simulink model "mod"  (R2019a)
settings: Solver=VariableStepAuto  StartTime=0  StopTime=1369  RelTol=1e-3
undefined symbols (not defined in the file): Ion, Lithium
libraries: nesl_utility x7, fl_lib x6, sdl_lib x5, autolibshared x4, ee_lib x3, powerlib x2, electricdrivelib x1
settings Model: SnapshotBufferSize=50  Creator=rachad  LastModifiedBy=rachad
settings GRTTargetCC: ExtMode=on

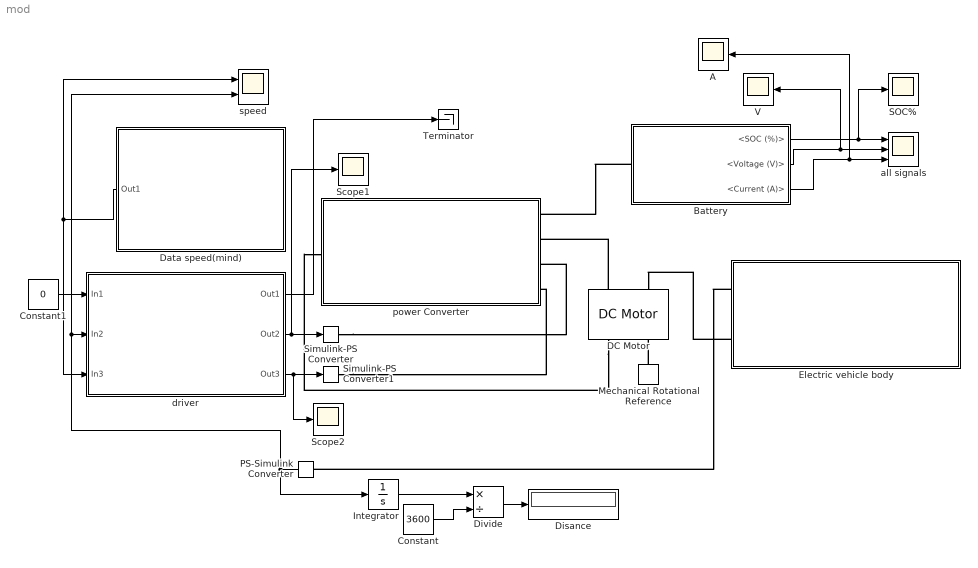
== system mod ==
  A : Scope
  Battery : Subsystem
  Constant : Constant  Value=3600
  Constant1 : Constant  Value=0
  DC Motor : ee_lib/Electromechanical/Brushed Motors/DC Motor  parameterization=3  Ra=3.9 Ohm  La=12e-6 H  emf_or_torque=1  Kv=0.072e-3 V/rpm  Ki=6.876e-4 N*m/A  T_stall=0.24e-3 N*m  w_max=15000 rpm  w_rated=12000 rpm  P_rated=150 kW  V_rated=300 V  J=0.01 g*cm^2  lam_param=1  lam=0 N*m/(rad/s)  i_noload=0 A  V_i_noload=1.5 V  speed0=0 rpm  alpha=3.93e-3 1/K  Tmeas=25 degC  thermal_mass=100 J/K  initial_temperature=25 degC
      settings: SourceProductName=Simscape Electrical
  Data speed(mind) : Subsystem
  Disance : Display
  Divide : Product  Inputs=*/
  Electric vehicle body : Subsystem
  Integrator : Integrator
  Mechanical Rotational Reference : fl_lib/Mechanical/Rotational Elements/Mechanical Rotational Reference
  PS-Simulink Converter : nesl_utility/PS-Simulink Converter  PhysicalDomain=network_engine_domain  SubClassName=ps_output  LeftPortType=input  RightPortType=output  PseudoPeriodic=off  Frequencies=[]  Unit=m/s  AffineConversion=off
  SOC% : Scope
  Scope1 : Scope
  Scope2 : Scope
  Simulink-PS Converter : nesl_utility/Simulink-PS Converter  PhysicalDomain=network_engine_domain  SubClassName=ps_input  LeftPortType=input  RightPortType=output  PseudoPeriodic=off  Frequencies=[]  NoiseDistribution=none  NoiseParameters=[]  Unit=1  AffineConversion=off  FilteringAndDerivatives=provide  SimscapeFilterOrder=1  InputFilterTimeConstant=0.001  UdotUserProvided=0
  Simulink-PS Converter1 : nesl_utility/Simulink-PS Converter  PhysicalDomain=network_engine_domain  SubClassName=ps_input  LeftPortType=input  RightPortType=output  PseudoPeriodic=off  Frequencies=[]  NoiseDistribution=none  NoiseParameters=[]  Unit=1  AffineConversion=off  FilteringAndDerivatives=provide  SimscapeFilterOrder=1  InputFilterTimeConstant=0.001  UdotUserProvided=0
  Terminator : Terminator
  V : Scope
  all signals : Scope  NumInputPorts=3
  driver : Subsystem
  power Converter : Subsystem
  speed : Scope  NumInputPorts=2
  wires:
  Divide/1 -> Disance/1
  Constant/1 -> Divide/2
  Integrator/1 -> Divide/1
  driver/2(Out2) -> Simulink-PS Converter/1, Scope1/1
  Constant1/1 -> driver/1(In1)
  driver/3(Out3) -> Simulink-PS Converter1/1, Scope2/1
  Data speed(mind)/1(Out1) -> speed/1, driver/3(In3)
  Battery/1(<SOC (%)>) -> SOC%/1, all signals/1
  Battery/2(<Voltage (V)>) -> V/1, all signals/2
  Battery/3(<Current (A)>) -> A/1, all signals/3
  PS-Simulink Converter/1 -> speed/2, driver/2(In2), Integrator/1
  driver/1(Out1) -> Terminator/1
  connections:
  Electric vehicle body/LConn2 -- DC Motor/LConn2
  Mechanical Rotational Reference/LConn1 -- DC Motor/RConn2
  Electric vehicle body/LConn1 -- PS-Simulink Converter/LConn1
  DC Motor/LConn1 -- power Converter/RConn2
  DC Motor/RConn1 -- power Converter/LConn1
  Simulink-PS Converter/RConn1 -- power Converter/RConn3
  Simulink-PS Converter1/RConn1 -- power Converter/RConn4
  Battery/LConn1 -- power Converter/RConn1

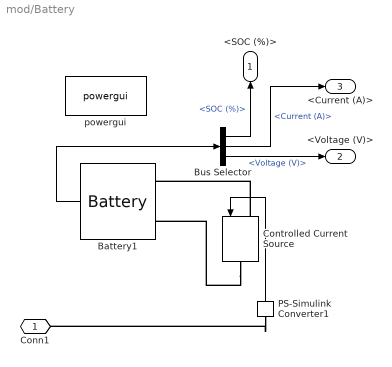
== system mod/Battery ==
  Battery1 : electricdrivelib/Extra Sources/Battery  BatType=Lithium-Ion  ShowTempParam=off  ThermalPreset=no  ShowAgeParam=off  NomV=300  NomQ=50  SOC=100  Batt_Tr=1  PresetModel=on  MaxQ=50  MinV=225  FullV=349.1961  Dis_rate=21.7391  R=0.06  Normal_OP=45.2174  expZone="[324.1158      2.456522]"  current=[6.5 13 32.5]  Units=Time  Tci=20  NomT=20  T2=-30  MaxQ2=4.8  FullV2=7.1  Normal_OP2=5.655  expZone2="[6.58           1]"  Rca=0.6  ti=2000  Dp=0  Neq0=0  Tsim=1e6  Ta1=25  Qeol=5.4*0.9  Reol=0.013333*1.2  Char_age=[2.3478, 3]  Dis_age=[2.3478, 10]  N1=1500  N2=10500  N3=1000  N4=1400  Ta2=45  N5=950
      settings: SourceProductName=Simscape Electrical
  Bus Selector : BusSelector  OutputSignals=SOC (%),Current (A),Voltage (V)
  Controlled Current Source : powerlib/Electrical Sources/Controlled Current Source  Initialize=off  Source_Type=DC  Amplitude=0  Phase=0  Frequency=0  Measurements=None
      settings: SourceProductName=Simscape Electrical
  PS-Simulink Converter1 : nesl_utility/PS-Simulink Converter  PhysicalDomain=network_engine_domain  SubClassName=ps_output  LeftPortType=input  RightPortType=output  PseudoPeriodic=off  Frequencies=[]  Unit=1  AffineConversion=off
  powergui : powerlib/powergui  Priority=1  SimulationMode=Continuous  SampleTime=50e-6  frequency=60  Iterations=50  frequencyindice=0  Pbase=100e6  ErrMax=1e-4  UnitsV=kV  UnitsW=MW  buscounter=0  FunctionMessages=off  echomessages=off  EnableUseOfTLC=off  CurrentSourceSwitches=off  DisableSnubberDevices=off  DisableRonSwitches=off  DisableVfSwitches=off  DisplayEquations=off  AutomaticDiscreteSolvers=off  SolverType=Tustin/Backward Euler (TBE)  Interpol=off  ExternalGateDelay=off  methode=off  Ts=100  x0status=blocks  SPID=on  SwTol=0  HookPort=off  NonlinearTolerance=0  nMaxIteration=15  ContinueOnMaxIteration=off  RestoreLinks=warning  ResistiveCurrentMeasurement=off  Frange=[0:2:500]  Ylog=off  Xlog=on  ShowGrid=off  save=off  variable=ZData  structure=0  ZoomFFT=off  StartTime=0.0  cycles=1  DisplayStyle=1  fundamental=60  FreqAxis=off  MaxFrequency=1000  frequencyindicesteady=1  RmsSteady=1  display=off
      settings: SourceProductName=Simscape Electrical
  Conn1 : PMIOPort  Side=Left
  <SOC (%)> : Outport
  <Voltage (V)> : Outport  Port=2
  <Current (A)> : Outport  Port=3
  wires:
  Bus Selector/2 -> <Current (A)>/1  "<Current (A)>"
  Bus Selector/3 -> <Voltage (V)>/1  "<Voltage (V)>"
  PS-Simulink Converter1/1 -> Controlled Current Source/1
  Battery1/1 -> Bus Selector/1
  Bus Selector/1 -> <SOC (%)>/1  "<SOC (%)>"
  connections:
  Controlled Current Source/LConn1 -- Battery1/LConn1
  Controlled Current Source/RConn1 -- Battery1/LConn2
  PS-Simulink Converter1/LConn1 -- Conn1/RConn1

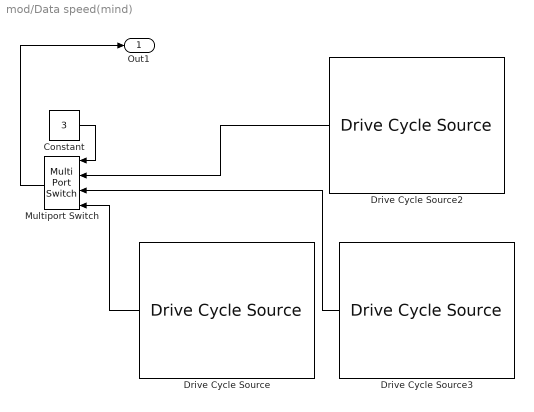
== system mod/Data speed(mind) ==
  Constant : Constant  Value=3
  Drive Cycle Source : autolibshared/Drive Cycle Source  cycleVar=.mat, .xls, .xlsx or .txt file  fileVar=C:\Users\rachad\Desktop\udds.txt  tfinal="1369  seconds"  cycleRepeat=off  outAccPort=off  outGearPort=off  gearList=No gear data  t_wot1=5  xdot_woto=0  xdot_wot1=30  t_wot2=20  xdot_wot2=0  t_wotend=30  srcUnit=m/s  outUnit=m/s  srcAccUnit=m/s/s  outAccUnit=m/s^2  dt=0  aMode=1
      settings: SourceProductName=Powertrain Blockset  SourceProductBaseCode=PW
  Drive Cycle Source2 : autolibshared/Drive Cycle Source  cycleVar=FTP75  fileVar=cycleFTP75.mat  tfinal="2474  seconds"  cycleRepeat=off  outAccPort=off  outGearPort=off  gearList=No gear data  t_wot1=5  xdot_woto=0  xdot_wot1=30  t_wot2=20  xdot_wot2=0  t_wotend=30  srcUnit=m/s  outUnit=m/s  srcAccUnit=m/s/s  outAccUnit=m/s^2  dt=0  aMode=1
      settings: SourceProductName=Powertrain Blockset  SourceProductBaseCode=PW
  Drive Cycle Source3 : autolibshared/Drive Cycle Source  cycleVar=.mat, .xls, .xlsx or .txt file  fileVar=C:\Users\rachad\Desktop\IM240.txt  tfinal="240  seconds"  cycleRepeat=off  outAccPort=off  outGearPort=off  gearList=No gear data  t_wot1=5  xdot_woto=0  xdot_wot1=30  t_wot2=20  xdot_wot2=0  t_wotend=30  srcUnit=m/s  outUnit=m/s  srcAccUnit=m/s/s  outAccUnit=m/s^2  dt=0  aMode=1
      settings: SourceProductName=Powertrain Blockset  SourceProductBaseCode=PW
  Multiport Switch : MultiPortSwitch
  Out1 : Outport
  wires:
  Multiport Switch/1 -> Out1/1
  Drive Cycle Source/1 -> Multiport Switch/4
  Constant/1 -> Multiport Switch/1
  Drive Cycle Source2/1 -> Multiport Switch/2
  Drive Cycle Source3/1 -> Multiport Switch/3

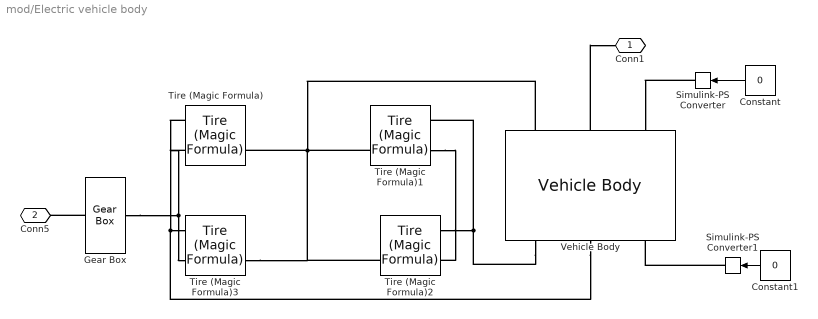
== system mod/Electric vehicle body ==
  Constant : Constant  Value=0
  Constant1 : Constant  Value=0
  Gear Box : fl_lib/Mechanical/Mechanisms/Gear Box  ratio=7  t_in_specify=off  t_in_priority=None  t_in=0 N*m  t_in_nominal_specify=off  t_in_nominal_unit=N*m  t_in_nominal_value=1  t_out_specify=off  t_out_priority=None  t_out=0 N*m  t_out_nominal_specify=off  t_out_nominal_unit=N*m  t_out_nominal_value=1
  Simulink-PS Converter : nesl_utility/Simulink-PS Converter  PhysicalDomain=network_engine_domain  SubClassName=ps_input  LeftPortType=input  RightPortType=output  PseudoPeriodic=off  Frequencies=[]  NoiseDistribution=none  NoiseParameters=[]  Unit=1  AffineConversion=off  FilteringAndDerivatives=provide  SimscapeFilterOrder=1  InputFilterTimeConstant=0.001  UdotUserProvided=0
  Simulink-PS Converter1 : nesl_utility/Simulink-PS Converter  PhysicalDomain=network_engine_domain  SubClassName=ps_input  LeftPortType=input  RightPortType=output  PseudoPeriodic=off  Frequencies=[]  NoiseDistribution=none  NoiseParameters=[]  Unit=1  AffineConversion=off  FilteringAndDerivatives=provide  SimscapeFilterOrder=1  InputFilterTimeConstant=0.001  UdotUserProvided=0
  Tire (Magic Formula){,1..3} (4 alike) : sdl_lib/Tires & Vehicles/Tire (Magic Formula)  parameterization=sdl.enum.magic_tire_model.peak  F_z1=3000 N  F_x1=3500 N  kappa1=10  B_m=10  C_m=1.9  D_m=1  E_m=0.97  fz0=4000 N  p_Cx=1.685  p_Dx=[1.21, -.037]  p_Ex=[.344, .095, -.02, 0]  p_Kx=[21.51, -.163, .245]  p_Hx=[-.002, .002]  p_Vx=[0, 0]  v_tr_thr=0.1 m/s  r_e=0.3 m  model_compliance=1  stiffness=1e6 N/m  damping=1000 N/(m/s)  model_inertia=0  inertia=1 kg*m^2  initial_velocity=0 rad/s  model_resistance=1  resistance_model=1  coeff=0.015  p_tire=250e3 Pa  alpha=-0.003  beta=0.97  coeff_a=84e-4  coeff_b=6.2e-4 s/m  coeff_c=1.6e-4 s^2/m^2  v_thr=0.001 m/s
      settings: SourceProductName=Simscape Driveline
  Vehicle Body : sdl_lib/Tires & Vehicles/Vehicle Body  mass=800 kg  n_w=2  x_f=1.4 m  x_r=1.6 m  y_c=0.5 m  mass_var=simscape.enum.onoff.off  model_pitch=simscape.enum.onoff.on  inertia=4000 kg*m^2  suspension_model=sdl.enum.linearTLU.linear  k_f=1e4 N/m  b_f=1e4 N/(m/s)  k_r=1e4 N/m  b_r=1e4 N/(m/s)  k_f_TLU=[-2000, -1000, 0, 1000, 2000] N  x_f_TLU=[-.4, -.2, 0, .2, .4] m  b_f_TLU=[-200, -100, 0, 100, 200] N  v_f_TLU=[-4, -2, 0, 2, 4] m/s  k_r_TLU=[-2000, -1000, 0, 1000, 2000] N  x_r_TLU=[-.4, -.2, 0, .2, .4] m  b_r_TLU=[-200, -100, 0, 100, 200] N  v_r_TLU=[-4, -2, 0, 2, 4] m/s  interp_method=simscape.enum.interpolation.linear  extrap_method=simscape.enum.extrapolation.linear  model_hardstop=simscape.enum.onoff.off  upper_bound_f=.25 m  lower_bound_f=-.25 m  stop_k_f=1e6 N/m  stop_b_f=150 N/(m/s)  upper_bound_r=.25 m  lower_bound_r=-.25 m  stop_k_r=1e6 N/m  stop_b_r=150 N/(m/s)  initial_pitch=0 rad  initial_pitch_rate=0 rad/s  g=9.81 m/s^2  liftoff_warning=simscape.enum.onoff.off  area=3 m^2  Cd=0.4  rho=1.18 kg/m^3  v_specify=off  v_priority=High  v=0 m/s  v_nominal_specify=off  v_nominal_unit=m/s  v_nominal_value=1
      settings: SourceProductName=Simscape Driveline
  Conn1 : PMIOPort  Side=Left
  Conn5 : PMIOPort  Port=2  Side=Left
  wires:
  Constant/1 -> Simulink-PS Converter/1
  Constant1/1 -> Simulink-PS Converter1/1
  connections:
  Tire (Magic Formula)1/RConn2 -- Tire (Magic Formula)2/RConn2 -- Tire (Magic Formula)3/RConn2 -- Vehicle Body/LConn1 -- Tire (Magic Formula)/RConn2
  Vehicle Body/RConn2 -- Tire (Magic Formula)/LConn1 -- Tire (Magic Formula)3/LConn1
  Tire (Magic Formula)/LConn2 -- Gear Box/RConn1 -- Tire (Magic Formula)3/LConn2
  Tire (Magic Formula)1/LConn2 -- Tire (Magic Formula)2/LConn2
  Vehicle Body/LConn2 -- Conn1/RConn1
  Vehicle Body/RConn1 -- Tire (Magic Formula)2/LConn1 -- Tire (Magic Formula)1/LConn1
  Gear Box/LConn1 -- Conn5/RConn1
  Simulink-PS Converter/RConn1 -- Vehicle Body/LConn3
  Simulink-PS Converter1/RConn1 -- Vehicle Body/RConn3

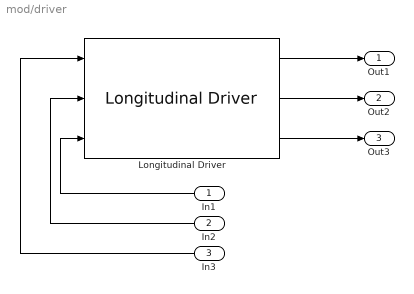
== system mod/driver ==
  In1 : Inport
  In2 : Inport  Port=2
  In3 : Inport  Port=3
  Longitudinal Driver : autolibshared/Longitudinal Driver  cntrlType=Scheduled PI  shftType=None  velUnits=m/s  gearOut=off  Kp=15  Ki=1  Kff=.05  Kg=.01  VehVelVec=[0 100]  KffVec=[.1 .1]  KpVec=[10 10]  KiVec=[5 5]  KgVec=[0 0]  m=1500  Kpt=3000  tau=.1  L=2  aR=200  bR=2.5  cR=.5  g=9.81  vnom=100  Kaw=.1  tauerr=.03  tauPt=2  GearInit=0  tShift=.1  pdlVec=[0.1 0.4 0.5 0.9]  upShftTbl=[-1 12.9375 26.4375 39.9375 51.18749999999999 62.4375 72.84375 83.25;-1 16.3125 29.8125 43.3125 54.5624 65.8125 76.78125 87.75;-1 19.6875 33.1875 46.68749999999999 57.9375 69.1875 80.71875 92.25;-1 33 52.5 77.25 100.5 138.75 161.875 185]  dwnShftTbl=[1 9.5625 23.0625 36.5625 47.8125 59.0625 68.90625 78.75;1 12.9375 26.4375 39.9375 51.18749999999999 62.4375 72.84375 83.25;1 16.3125 29.8125 43.3125 54.562499 65.8125 76.78125 87.75;1 19.6875 33.1875 46.68749999999999 57.9375 69.1875 80.71875 92.25]  tClutch=.5  tRev=.5  tPark=120  aMode=1  UpGearVec="[0  1  2  3  4  5  6  7]"  DownGearVec="[1  2  3  4  5  6  7  8]"
      settings: SourceProductName=Powertrain Blockset  SourceProductBaseCode=PW
  Out1 : Outport
  Out2 : Outport  Port=2
  Out3 : Outport  Port=3
  wires:
  Longitudinal Driver/2 -> Out2/1
  In3/1 -> Longitudinal Driver/1
  Longitudinal Driver/1 -> Out1/1
  In2/1 -> Longitudinal Driver/2
  In1/1 -> Longitudinal Driver/3
  Longitudinal Driver/3 -> Out3/1

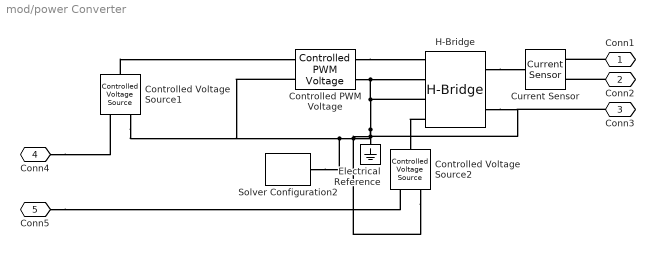
== system mod/power Converter ==
  Controlled PWM Voltage : ee_lib/Integrated Circuits/Controlled PWM Voltage  F=1000 Hz  TD=0 s  pulse_width_offset=0 s  pulse_min=0 s  Vmin=0 V  Vmax=5 V  Vm=60 V  pwm_or_av=2  event_type=1  sample_time=1e-6 s  u_min=0  u_max=1
      settings: SourceProductName=Simscape Electrical
  Controlled Voltage Source1 : fl_lib/Electrical/Electrical Sources/Controlled Voltage Source
  Controlled Voltage Source2 : fl_lib/Electrical/Electrical Sources/Controlled Voltage Source
  Current Sensor : fl_lib/Electrical/Electrical Sensors/Current Sensor
  Electrical Reference : fl_lib/Electrical/Electrical Elements/Electrical Reference
  H-Bridge : ee_lib/Semiconductors & Converters/Converters/H-Bridge  Venable=2.5 V  Vmax=5.0 V  Vreverse=2.5 V  Vbrake=2.5 V  Vm=300 V  pwm_or_av=2  discontinuous=0  freewheeling_mode=1  freewheeling_mode_disc=1  Ron=0.1 Ohm  Don=0.05 Ohm  Rload=10 Ohm  Lload=1e-5 H  F=10 kHz  thermal_mass=100 J/K  initial_temperature=298.15 K  Ron2=0.1 Ohm  Don2=0.05 Ohm  Tmeas=298.15 K  Tmeas2=398.15 K
      settings: SourceProductName=Simscape Electrical
  Solver Configuration2 : nesl_utility/Solver Configuration  PhysicalDomain=network_engine_domain  SubClassName=solver  LeftPortType=input  RightPortType=generic  Tones=[]  Harmonics=[]  SimulateNoise=off  Profile=off  UseLocalSampling=off  EnableSwitchedLinearOptims=on  FrequencyDomain=off  UseCCode=off  RelTol=0.001  AbsTol=1e-06  MinStep=1e-09  ToWorkspace=off  RevertToSquareIcSolve=off  NumHomotopyIterations=100  PhasorMode=off  PhasorModeNumHarmonics=1  DoDC=off  ResidualTolerance=1e-09  UseLocalSolver=off  LocalSolverChoice=NE_BACKWARD_EULER_ADVANCER  LocalSolverSampleTime=0.001  DoFixedCost=off  MaxNonlinIter=3  MaxModeIter=2  LinearAlgebra=auto  EquationFormulation=NE_TIME_EF  DelaysMemoryBudget=1024  AutomaticFiltering=on  FilteringTimeConstant=0.001  PartitionStorageMethod=AS_NEEDED  PartitionMemoryBudget=1024  PartitionMethod=ROBUST
  Conn1 : PMIOPort  Side=Right
  Conn2 : PMIOPort  Port=2  Side=Right
  Conn3 : PMIOPort  Port=3  Side=Left
  Conn4 : PMIOPort  Port=4  Side=Right
  Conn5 : PMIOPort  Port=5  Side=Right
  connections:
  Conn2/RConn1 -- Current Sensor/RConn2
  Conn4/RConn1 -- Controlled Voltage Source1/RConn1
  H-Bridge/LConn4 -- Controlled Voltage Source2/LConn1
  H-Bridge/LConn3 -- H-Bridge/LConn2 -- Controlled PWM Voltage/RConn2 -- H-Bridge/RConn2 -- Conn3/RConn1 -- Controlled Voltage Source2/RConn2 -- Controlled PWM Voltage/LConn2 -- Controlled Voltage Source1/RConn2 -- Solver Configuration2/RConn1 -- Electrical Reference/LConn1
  Controlled Voltage Source1/LConn1 -- Controlled PWM Voltage/LConn1
  H-Bridge/RConn1 -- Current Sensor/LConn1
  Conn5/RConn1 -- Controlled Voltage Source2/RConn1
  Controlled PWM Voltage/RConn1 -- H-Bridge/LConn1
  Conn1/RConn1 -- Current Sensor/RConn1
